simulink model "PV_MPPT_v1_before_phase1_fix"  (R2025a)
settings: Solver=VariableStepAuto  StartTime=0.0  StopTime=1  RelTol=1e-3
undefined symbols (not defined in the file): Ion, Lithium
libraries: spsSeriesRLCBranchLib x7, spsCurrentMeasurementLib x3, spsIGBTDiodeLib x3, spsVoltageMeasurementLib x2, spsBatteryLib x1, spsDiodeLib x1, spsControlledCurrentSourceLib x1, spsPVArrayLib x1, sps_lib x1
settings Model: Creator=Limingyu  LastModifiedBy=Limingyu

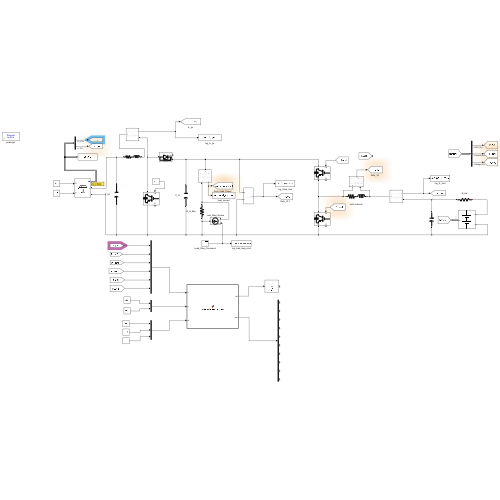
[thumbnail: Simulink's stored preview of the top-level diagram]
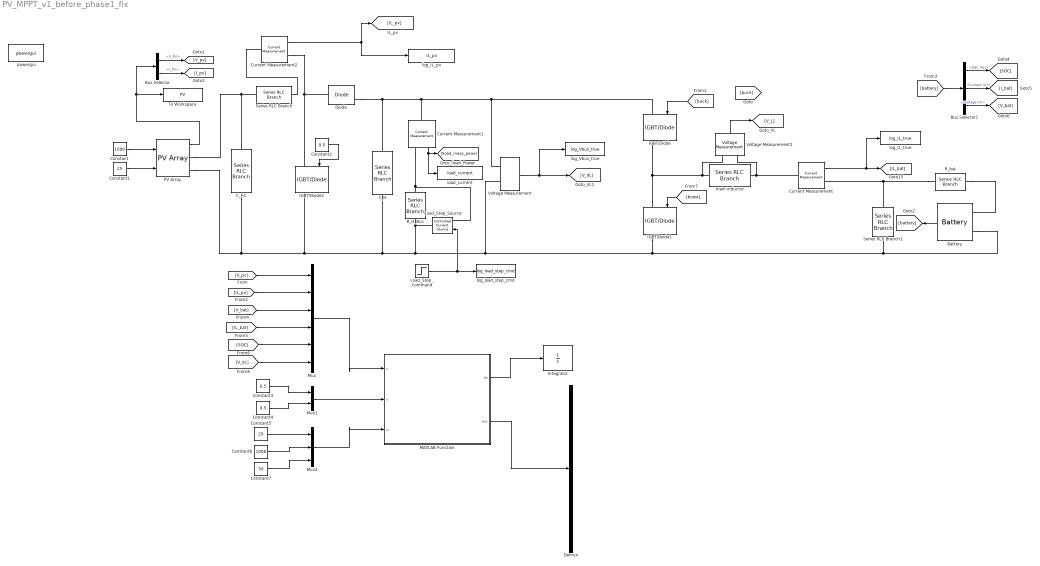
== system PV_MPPT_v1_before_phase1_fix ==
  Battery : spsBatteryLib/Battery  BatType=Lithium-Ion  NomV=300  NomQ=20  SOC=80  Batt_Tr=30  PresetModel=on  MaxQ=20  MinV=225  FullV=349.1961  Dis_rate=8.6957  R=0.15  Normal_OP=18.087  expZone="[324.1158     0.9826087]"
  Bus Selector : BusSelector  OutputSignals=V_PV,I_PV
  Bus Selector1 : BusSelector  OutputSignals=SOC (%),Current (A),Voltage (V)
  C_H : spsSeriesRLCBranchLib/Series RLC Branch  LConnTagsString=__new0  RConnTagsString=__new0  BranchType=C  Resistance=50  Inductance=1e-3  SetiL0=off  InitialCurrent=0  Capacitance=1500e-6  Setx0=on  InitialVoltage=600  Measurements=Branch voltage
  C_H1 : spsSeriesRLCBranchLib/Series RLC Branch  LConnTagsString=__new0  RConnTagsString=__new0  BranchType=C  Resistance=200  Inductance=1e-3  SetiL0=off  InitialCurrent=0  Capacitance=300e-6  Setx0=on  InitialVoltage=600  Measurements=Branch voltage
  Constant : Constant  Value=1000
  Constant1 : Constant  Value=25
  Constant2 : Constant  Value=0.5
  Constant3 : Constant  Value=0.5
  Constant4 : Constant  Value=0.5
  Constant5 : Constant  Value=25
  Constant6 : Constant  Value=1000
  Constant7 : Constant  Value=50
  Current Measurement : spsCurrentMeasurementLib/Current Measurement  PhasorSimulation=off  OutputType=Complex  PSBequivalent=0
  Current Measurement1 : spsCurrentMeasurementLib/Current Measurement  PhasorSimulation=off  OutputType=Complex  PSBequivalent=0
  Current Measurement2 : spsCurrentMeasurementLib/Current Measurement  PhasorSimulation=off  OutputType=Complex  PSBequivalent=0
  Demux : Demux  Outputs=10
  Diode : spsDiodeLib/Diode  Ron=0.001  Lon=0  Vf=0.8  IC=0  UseSnubber=0  Rs=500  Cs=250e-9  Measurements=on
  IGBT/Diode : spsIGBTDiodeLib/IGBT//Diode  Ron=1e-3  Rs=1e5  Cs=inf  Measurements=on
  IGBT/Diode1 : spsIGBTDiodeLib/IGBT//Diode  Ron=1e-3  Rs=1e5  Cs=inf  Measurements=on
  IGBT/Diode2 : spsIGBTDiodeLib/IGBT//Diode  Ron=1e-3  Rs=1e5  Cs=inf  Measurements=on
  Integrator : Integrator
  Load_Step_Command : Step  Time=0  After=0  SampleTime=1e-6
  Load_Step_Source : spsControlledCurrentSourceLib/Controlled Current Source  Initialize=on  Source_Type=AC  Amplitude=0  Phase=0  Frequency=0  Measurements=None
  MATLAB Function : MATLAB Function  TreatAsAtomicUnit=on
  Mux : Mux  Inputs=6
  Mux1 : Mux  Inputs=2
  Mux2 : Mux  Inputs=3
  PV Array : spsPVArrayLib/PV Array  Npar=9  Nser=5  PlotType=array @ 1000 W/m2 & specified temperatures  S_vec="[ 1000  500  100 ]"  Temp_C_vec="[ 45 25  ]"  ModuleName=User-defined  PlotWhenSelected=off  Pm=213.15  Ncell=60  Voc=36.3  Isc=7.84  Vm=29  Im=7.35  beta_Voc_pc=-0.36099  alpha_Isc_pc=0.102  beta_Voc=-0.13104  alpha_Isc=0.0079968  IL=7.8654  I0=2.9273e-10  nI=0.98119  Rsh=313.0553  Rs=0.39381  RobustModel=off  RobustCellTemperature=313.3991  BAL=on  Tc=1e-6  Tfilter=5e-5
  R_H_Bus : spsSeriesRLCBranchLib/Series RLC Branch  LConnTagsString=__new0  RConnTagsString=__new0  BranchType=R  Resistance=50  Inductance=1e-3  SetiL0=off  InitialCurrent=0  Capacitance=1e-6  Setx0=off  InitialVoltage=0  Measurements=None
  R_bat : spsSeriesRLCBranchLib/Series RLC Branch  LConnTagsString=__new0  RConnTagsString=__new0  BranchType=R  Resistance=0.05  Inductance=1e-3  SetiL0=off  InitialCurrent=0  Capacitance=1e-6  Setx0=off  InitialVoltage=0  Measurements=None
  Series RLC Branch : spsSeriesRLCBranchLib/Series RLC Branch  LConnTagsString=__new0  RConnTagsString=__new0  BranchType=RL  Resistance=10e-3  Inductance=10e-3  SetiL0=off  InitialCurrent=0  Capacitance=1e-6  Setx0=off  InitialVoltage=0  Measurements=Branch current
  Series RLC Branch1 : spsSeriesRLCBranchLib/Series RLC Branch  LConnTagsString=__new0  RConnTagsString=__new0  BranchType=C  Resistance=1  Inductance=1e-3  SetiL0=off  InitialCurrent=0  Capacitance=300e-3  Setx0=on  InitialVoltage=300  Measurements=None
  To Workspace : ToWorkspace  VariableName=PV  SaveFormat=Timeseries  SampleTime=-1
  Voltage Measurement : spsVoltageMeasurementLib/Voltage Measurement  PhasorSimulation=off  OutputType=Complex  PSBequivalent=0
  Voltage Measurement2 : spsVoltageMeasurementLib/Voltage Measurement  PhasorSimulation=off  OutputType=Complex  PSBequivalent=0
  load_current : ToWorkspace  VariableName=load_current  SaveFormat=Timeseries  SampleTime=-1
  log_IL_pv : ToWorkspace  VariableName=IL_pv  SaveFormat=Timeseries  SampleTime=-1
  log_IL_true : ToWorkspace  VariableName=log_IL_true  SaveFormat=Timeseries  SampleTime=-1
      settings: Decimation=20
  log_Vbus_true : ToWorkspace  VariableName=log_Vbus_true  SaveFormat=Timeseries  SampleTime=-1
      settings: Decimation=20
  log_load_step_cmd : ToWorkspace  VariableName=log_load_step_cmd  SaveFormat=Timeseries  SampleTime=-1
      settings: Decimation=20
  main inductor : spsSeriesRLCBranchLib/Series RLC Branch  LConnTagsString=__new0  RConnTagsString=__new0  BranchType=RL  Resistance=10e-3  Inductance=10e-3  SetiL0=off  InitialCurrent=0  Capacitance=1e-6  Setx0=off  InitialVoltage=0  Measurements=None
  powergui : sps_lib/powergui  Priority=1  SimulationMode=Discrete  SampleTime=10e-6  frequency=60  Iterations=50  frequencyindice=0  Pbase=100e6  ErrMax=1e-4  UnitsV=kV  UnitsW=MW  buscounter=0  FunctionMessages=off  echomessages=off  EnableUseOfTLC=off  CurrentSourceSwitches=off  DisableSnubberDevices=off  DisableRonSwitches=off  DisableVfSwitches=off  DisplayEquations=off  AutomaticDiscreteSolvers=off  SolverType=Tustin/Backward Euler (TBE)  Interpol=off  ExternalGateDelay=off  methode=off  Ts=100  x0status=blocks  SPID=on  SwTol=0  HookPort=off  NonlinearTolerance=1e-4  nMaxIteration=100  ContinueOnMaxIteration=off  RestoreLinks=warning  ResistiveCurrentMeasurement=off  Frange=[0:2:500]  Ylog=off  Xlog=on  ShowGrid=off  save=off  variable=ZData  structure=0  ZoomFFT=off  StartTime=0.0  cycles=1  DisplayStyle=1  fundamental=60  FreqAxis=off  MaxFrequency=1000  frequencyindicesteady=1  RmsSteady=1  display=off
  wires:
  [buck] -> IGBT/Diode/1
  Load_Step_Command/1 -> log_load_step_cmd/1, Load_Step_Source/1
  Voltage Measurement/1 -> [V_dc], log_Vbus_true/1
  Current Measurement1/1 -> load_current/1, [Iload_meas_power]
  Battery/1 -> [battery]
  Voltage Measurement2/1 -> [V_L]
  [boost] -> IGBT/Diode1/1
  Current Measurement/1 -> [IL_bat], log_IL_true/1
  PV Array/1 -> Bus Selector/1, To Workspace/1
  Constant/1 -> PV Array/1
  Constant1/1 -> PV Array/2
  Mux/1 -> MATLAB Function/1(x)
  Bus Selector/1 -> [V_pv]  "<V_PV>"
  Bus Selector/2 -> [I_pv]  "<I_PV>"
  [V_pv] -> Mux/1
  Constant2/1 -> IGBT/Diode2/1
  Current Measurement2/1 -> log_IL_pv/1, [IL_pv]
  [IL_pv] -> Mux/2
  [battery] -> Bus Selector1/1
  Bus Selector1/1 -> [SOC]  "<SOC (%)>"
  Bus Selector1/2 -> [I_bat]  "<Current (A)>"
  Bus Selector1/3 -> [V_bat]  "<Voltage (V)>"
  [V_bat] -> Mux/3
  [IL_bat] -> Mux/4
  [SOC] -> Mux/5
  [V_dc] -> Mux/6
  Mux1/1 -> MATLAB Function/2(u)
  Constant3/1 -> Mux1/1
  Constant4/1 -> Mux1/2
  Mux2/1 -> MATLAB Function/3(w)
  Constant5/1 -> Mux2/1
  Constant6/1 -> Mux2/2
  Constant7/1 -> Mux2/3
  MATLAB Function/2(aux) -> Demux/1
  MATLAB Function/1(dx) -> Integrator/1
  connections:
  IGBT/Diode1/LConn1 -- IGBT/Diode/RConn1 -- Voltage Measurement2/LConn1 -- main inductor/LConn1
  Voltage Measurement/LConn1 -- IGBT/Diode/LConn1 -- Current Measurement1/LConn1 -- Diode/RConn1 -- C_H/LConn1
  R_H_Bus/LConn1 -- Current Measurement1/RConn1 -- Load_Step_Source/LConn1
  Voltage Measurement/LConn2 -- Battery/LConn2 -- Series RLC Branch1/RConn1 -- IGBT/Diode1/RConn1 -- PV Array/RConn2 -- C_H1/RConn1 -- IGBT/Diode2/RConn1 -- C_H/RConn1 -- R_H_Bus/RConn1 -- Load_Step_Source/RConn1
  main inductor/RConn1 -- Voltage Measurement2/LConn2 -- Current Measurement/LConn1
  R_bat/RConn1 -- Series RLC Branch1/LConn1 -- Current Measurement/RConn1
  R_bat/LConn1 -- Battery/LConn1
  PV Array/RConn1 -- C_H1/LConn1 -- Series RLC Branch/LConn1
  Diode/LConn1 -- Current Measurement2/RConn1 -- IGBT/Diode2/LConn1
  Series RLC Branch/RConn1 -- Current Measurement2/LConn1

== matlab function PV_MPPT_v1_before_phase1_fix/MATLAB Function ==
  data: x input; u input; dx output; w input; aux output
function [dx, aux] = Plant_Derivatives_Block(x, u, w)
%PLANT_DERIVATIVES_BLOCK Paste-ready code for a MATLAB Function block.
%   Inputs:
%     x = [vpv; iLpv; vb; iLb; SoC; vdc]
%     u = [dpv; db]
%     w = [temperature_degC; irradiance_Wm2; Rload_ohm]
%
%   Outputs:
%     dx  = six continuous-time state derivatives
%     aux = [Ipv; Ib; Ebat; dpv; db; Ppv; PpvBus; ...
%            PbatBus; Pload; powerBalanceResidual]
%
%   Current signs:
%     Ib > 0 and PbatBus > 0 mean battery discharge.
%     Ib < 0 and PbatBus < 0 mean battery charge.
%
%#codegen

%% Published converter and DC-bus parameters
Cpv = 300e-6;
Lpv = 10e-3;
rLpv = 10e-3;

Cb = 300e-6;
Lb = 10e-3;
rLb = 10e-3;

Cdc = 1500e-6;

%% Published battery ratings and phase-1 assumptions
batteryCapacityAh = 20;
batteryNominalVoltage = 300;
batteryInternalResistance = 0.05;  % Phase-1 assumption
batteryNominalSoC = 0.8;
batteryOcvSlope = 0;               % Constant OCV in phase 1

%% Published PV-module data
moduleVmp = 29;
moduleImp = 7.35;
moduleVoc = 36.3;
moduleIsc = 7.84;

%% Phase-1 PV-array and environmental assumptions
seriesModules = 9;
parallelStrings = 5;
referenceTemperatureC = 25;
referenceIrradiance = 1000;
iscTempCoefficient = 0.0005 * moduleIsc;
vocTempCoefficient = -0.0032 * moduleVoc;
vocLogCoefficient = 2.0;
minimumIrradianceRatio = 1e-6;

currentRatioAtMpp = moduleImp / moduleIsc;
voltageRatioAtMpp = moduleVmp / moduleVoc;
curveExponent = log(1 - currentRatioAtMpp) ...
    / log(voltageRatioAtMpp);

%% Unpack states, commands, and disturbances
vpv = x(1);
iLpv = x(2);
vb = x(3);
iLb = x(4);
soc = x(5);
vdc = x(6);

dpv = min(max(u(1), 0), 1);
db = min(max(u(2), 0), 1);

temperatureC = w(1);
irradiance = max(w(2), 0);
Rload = max(w(3), 1);

%% Empirical PV I-V curve
if irradiance <= 1e-6
    Ipv = 0;
else
    temperatureOffset = temperatureC - referenceTemperatureC;
    irradianceRatio = irradiance / referenceIrradiance;

    moduleIscNow = moduleIsc ...
        + iscTempCoefficient * temperatureOffset;
    arrayIsc = parallelStrings * irradianceRatio ...
        * max(moduleIscNow, 0);

    moduleVocNow = moduleVoc ...
        + vocTempCoefficient * temperatureOffset ...
        + vocLogCoefficient ...
        * log(max(irradianceRatio, minimumIrradianceRatio));
    moduleVocNow = max(moduleVocNow, 1);
    arrayVoc = seriesModules * moduleVocNow;

    normalizedVoltage = max(vpv, 0) / arrayVoc;
    if normalizedVoltage >= 1
        Ipv = 0;
    else
        Ipv = arrayIsc ...
            * (1 - normalizedVoltage^curveExponent);
    end
end

%% Simplified phase-1 battery model
boundedSoC = min(max(soc, 0), 1);
Ebat = batteryNominalVoltage ...
    + batteryOcvSlope * (boundedSoC - batteryNominalSoC);
Ib = (Ebat - vb) / batteryInternalResistance;

%% Six-state averaged plant equations
dx = zeros(6, 1);
dx(1) = (Ipv - iLpv) / Cpv;
dx(2) = (-rLpv * iLpv + vpv ...
    - (1 - dpv) * vdc) / Lpv;
dx(3) = (Ib - iLb) / Cb;
dx(4) = (-rLb * iLb + vb ...
    - (1 - db) * vdc) / Lb;

% Corrected form of the paper's Equation (12): SoC depends on battery
% current, equivalently on Ebat - vb, not on inductor current x(4).
dx(5) = -Ib / (3600 * batteryCapacityAh);

dx(6) = ((1 - dpv) * iLpv ...
    + (1 - db) * iLb ...
    - vdc / Rload) / Cdc;

%% Diagnostic outputs
Ppv = vpv * Ipv;
PpvBus = vdc * (1 - dpv) * iLpv;
PbatBus = vdc * (1 - db) * iLb;
Pload = vdc^2 / Rload;
dcBusStoredPower = Cdc * vdc * dx(6);
powerBalanceResidual = PpvBus + PbatBus ...
    - Pload - dcBusStoredPower;

aux = zeros(10, 1);
aux(1) = Ipv;
aux(2) = Ib;
aux(3) = Ebat;
aux(4) = dpv;
aux(5) = db;
aux(6) = Ppv;
aux(7) = PpvBus;
aux(8) = PbatBus;
aux(9) = Pload;
aux(10) = powerBalanceResidual;
end
